simulink model "lab_10_2"  (R2022b)
settings: Solver=VariableStepAuto  StartTime=0.0  StopTime=10  RelTol=1e-3
undefined symbols (not defined in the file): A, B, K, K1, K2, K3, Q, R
settings Model: Creator=osini  LastModifiedBy=osini

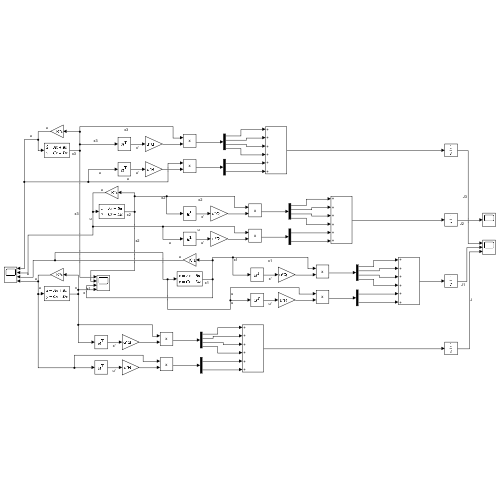
[thumbnail: Simulink's stored preview of the top-level diagram]
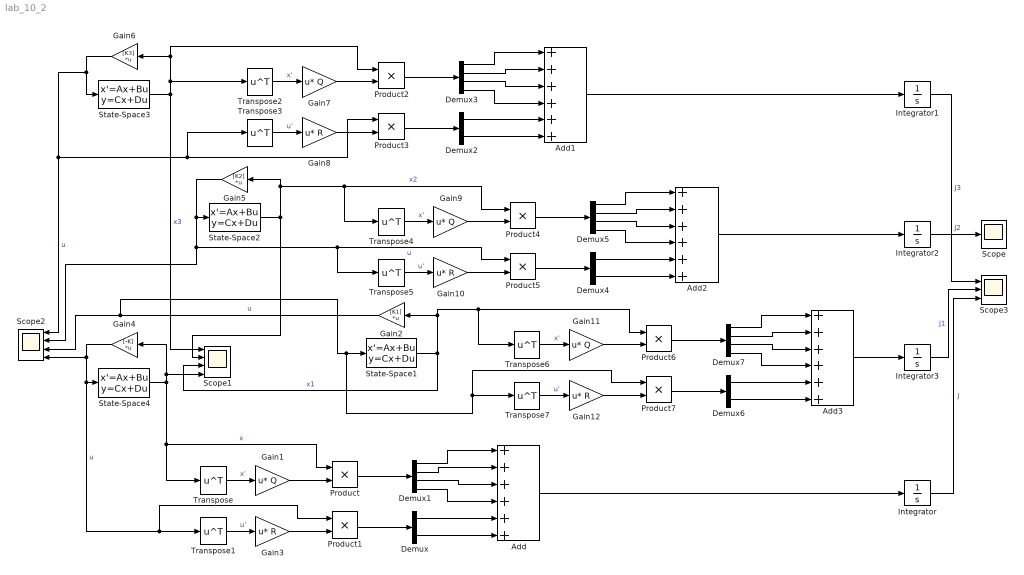
== system lab_10_2 ==
  Add{,1..3} (4 alike) : Sum  Inputs=++++++
  Demux{,2,4,6} (4 alike) : Demux  Outputs=2
  Demux{1,3,5,7} (4 alike) : Demux
  Gain{1,7,9,11} (4 alike) : Gain  Gain=Q  Multiplication=Matrix(u*K)
  Gain{3,8,10,12} (4 alike) : Gain  Gain=R  Multiplication=Matrix(u*K)
  Gain2 : Gain  Gain=[K1]  Multiplication=Matrix(K*u)
  Gain4 : Gain  Gain=[-K]  Multiplication=Matrix(K*u)
  Gain5 : Gain  Gain=[K2]  Multiplication=Matrix(K*u)
  Gain6 : Gain  Gain=[K3]  Multiplication=Matrix(K*u)
  Integrator{,1..3} (4 alike) : Integrator
  Product{,1..7} (8 alike) : Product
  Scope : Scope
  Scope1 : Scope  NumInputPorts=4
  Scope2 : Scope  NumInputPorts=4
  Scope3 : Scope  NumInputPorts=3
  State-Space{1..4} (4 alike) : StateSpace  A=A  B=B  C=eye(4)  D=zeros(4,2)  InitialCondition=1
  Transpose{,1..7} (8 alike) : Math  Operator=transpose
  wires:
  Add/1 -> Integrator/1
  Product/1 -> Demux1/1
  Demux1/1 -> Add/1
  Demux/1 -> Add/5
  State-Space4/1 -> Transpose/1, Product/1, Gain4/1, Scope1/4  "x"
  Integrator/1 -> Scope3/3  "J"
  Demux1/2 -> Add/2
  Demux1/4 -> Add/4
  Gain3/1 -> Product1/2
  Gain1/1 -> Product/2
  Gain4/1 -> Product1/1, Transpose1/1, State-Space4/1, Scope2/4  "u"
  Product1/1 -> Demux/1
  Transpose/1 -> Gain1/1  "x'"
  Demux/2 -> Add/6
  Transpose1/1 -> Gain3/1  "u'"
  Demux1/3 -> Add/3
  Transpose3/1 -> Gain8/1  "u'"
  Demux3/3 -> Add1/3
  Product3/1 -> Demux2/1
  Demux2/2 -> Add1/6
  Gain6/1 -> Transpose3/1, Product3/1, Scope2/1, State-Space3/1  "u"
  Transpose2/1 -> Gain7/1  "x'"
  Gain7/1 -> Product2/2
  Demux3/4 -> Add1/4
  Demux3/2 -> Add1/2
  Gain8/1 -> Product3/2
  State-Space3/1 -> Transpose2/1, Product2/1, Gain6/1, Scope1/1  "x3"
  Demux3/1 -> Add1/1
  Product2/1 -> Demux3/1
  Demux2/1 -> Add1/5
  Transpose5/1 -> Gain10/1  "u'"
  Demux5/3 -> Add2/3
  Product5/1 -> Demux4/1
  Demux4/2 -> Add2/6
  Gain5/1 -> Scope2/2, Transpose5/1, Product5/1, State-Space2/1  "u"
  Transpose4/1 -> Gain9/1  "x'"
  Gain9/1 -> Product4/2
  Demux5/4 -> Add2/4
  Demux5/2 -> Add2/2
  Gain10/1 -> Product5/2
  State-Space2/1 -> Transpose4/1, Product4/1, Gain5/1, Scope1/2  "x2"
  Demux5/1 -> Add2/1
  Product4/1 -> Demux5/1
  Demux4/1 -> Add2/5
  Add1/1 -> Integrator1/1
  Integrator1/1 -> Scope3/1  "J3"
  Add2/1 -> Integrator2/1
  Transpose7/1 -> Gain12/1  "u'"
  Demux7/3 -> Add3/3
  Product7/1 -> Demux6/1
  Demux6/2 -> Add3/6
  Gain2/1 -> Transpose7/1, Product7/1, State-Space1/1, Scope2/3  "u"
  Transpose6/1 -> Gain11/1  "x'"
  Gain11/1 -> Product6/2
  Demux7/4 -> Add3/4
  Demux7/2 -> Add3/2
  Gain12/1 -> Product7/2
  State-Space1/1 -> Transpose6/1, Product6/1, Gain2/1, Scope1/3  "x1"
  Demux7/1 -> Add3/1
  Product6/1 -> Demux7/1
  Demux6/1 -> Add3/5
  Add3/1 -> Integrator3/1
  Integrator3/1 -> Scope3/2  "J1"
  Integrator2/1 -> Scope/1  "J2"
